simulink model "Ej5"  (R2018a)
settings: Solver=VariableStepDiscrete  StartTime=0.0  StopTime=.5  RelTol=1e-3  EnableMultiTasking=on
libraries: dspstat3 x2, simulink_extras x1
settings Model: Creator=rcheng  LastModifiedBy=joses
settings DataIOCC: LimitDataPoints=on  SaveFormat=Array  SignalLoggingSaveFormat=ModelDataLogs
settings OptimizationCC: ExpressionDepthLimit=2147483647  InitFltsAndDblsToZero=on  LifeSpan=inf
settings DebuggingCC: UnderspecifiedInitializationDetection=Classic  MergeDetectMultiDrivingBlocksExec=none  SolverPrmCheckMsg=warning  FcnCallInpInsideContextMsg=warning  StateNameClashWarn=warning  SFUnexpectedBacktrackingDiag=warning  SFNoUnconditionalDefaultTransitionDiag=warning  SFExecutionAtInitializationDiag=none
settings HardwareCC: ProdBitPerPointer=32  ProdBitPerSizeT=32  ProdBitPerPtrDiffT=32  ProdLargestAtomicFloat=None  ProdIntDivRoundTo=Undefined  ProdEndianess=Unspecified  ProdWordSize=32  ProdHWDeviceType=32-bit Generic
settings ModelReferenceCC: PropagateSignalLabelsOutOfModel=off
settings CodeAppCC: StateflowObjectComments=on
settings GRTTargetCC: TargetLangStandard=C89/C90 (ANSI)  CombineOutputUpdateFcns=off  GRTInterface=on
settings ConfigComp: CovMetricSettings=dw  CovSaveCumulativeToWorkspaceVar=on  CovSaveSingleToWorkspaceVar=on  CovExternalEMLEnable=off  CovSFcnEnable=off

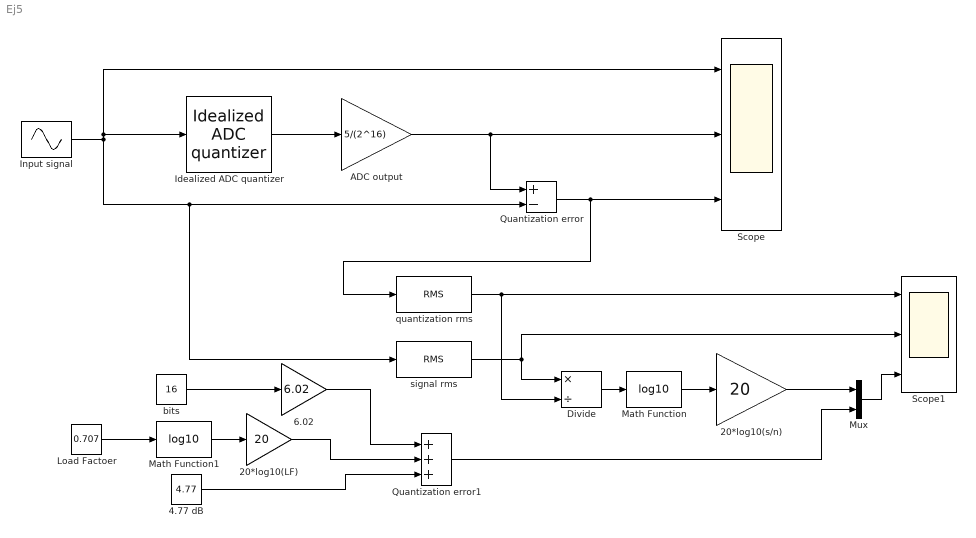
== system Ej5 ==
  20*log10(LF) : Gain  Gain=20
  20*log10(s/n) : Gain  Gain=20
  4.77 dB : Constant  Value=4.77
  6.02 : Gain  Gain=6.02
  ADC output : Gain  Gain=5/(2^16)
  Divide : Product  Inputs=*/  SaturateOnIntegerOverflow=on
  Idealized ADC quantizer : simulink_extras/Additional Discrete/Idealized ADC quantizer  NumberOfConverterBits=16  Vmin=-2.5  Vmax=2.5  OutputDataType=int16  OutputNegativeValues=on
      settings: SourceProductName=Simulink
  Input signal : Sin  Amplitude=2.5  Frequency=2*pi*100  SampleTime=1/10000
  Load Factoer : Constant  Value=0.707
  Math Function : Math  Operator=log10  SaturateOnIntegerOverflow=on
  Math Function1 : Math  Operator=log10  SaturateOnIntegerOverflow=on
  Mux : Mux  Inputs=2
  Quantization error : Sum  Inputs=+-
  Quantization error1 : Sum  Inputs=+++
  Scope : Scope  NumInputPorts=3
  Scope1 : Scope  NumInputPorts=3
  bits : Constant  Value=16
  quantization rms : dspstat3/RMS  run=on  directionMode=Each column  dimension=1  InputProcessing=Columns as channels (frame based)  reset_popup=None
  signal rms : dspstat3/RMS  run=on  directionMode=Each column  dimension=1  InputProcessing=Columns as channels (frame based)  reset_popup=None
  wires:
  Quantization error/1 -> Scope/3, quantization rms/1
  Idealized ADC quantizer/1 -> ADC output/1
  ADC output/1 -> Scope/2, Quantization error/1
  Input signal/1 -> Idealized ADC quantizer/1, Scope/1, signal rms/1, Quantization error/2
  quantization rms/1 -> Divide/2, Scope1/1
  signal rms/1 -> Divide/1, Scope1/2
  Math Function/1 -> 20*log10(s/n)/1
  Divide/1 -> Math Function/1
  20*log10(s/n)/1 -> Mux/1
  Mux/1 -> Scope1/3
  Load Factoer/1 -> Math Function1/1
  Math Function1/1 -> 20*log10(LF)/1
  Quantization error1/1 -> Mux/2
  bits/1 -> 6.02/1
  6.02/1 -> Quantization error1/1
  20*log10(LF)/1 -> Quantization error1/2
  4.77 dB/1 -> Quantization error1/3
